simulink model "ThdRwRtStFwdBkwdIsPosChk"  (R2018b)
settings: Solver=FixedStepDiscrete  StartTime=0.0  StopTime=10.0  FixedStep=0.01  RelTol=1e-3
undefined symbols (not defined in the file or in its folder): KeSMSuThirdRwStFwdBkwdPosDelta_Val, KeSMSuThirdRwStFwdBkwdPosTolr_Val, KeSMSuVehicleModelConfig_Val
libraries: StIsPosChkLib x11, simulink x5
(part 1 of 2)
settings Model: Creator=sn2xws  LastModifiedBy=sn55gm
settings Model: ModifiedHistory=|
  | 2024.1.24
  | bug695362 7s 调用模式VIP R，3R无响应
  | 2024.3.14
  | V2.5.0
  | Bug 813950 童锁Lock，Mode1_Easy Entry Mode 不应调用失败
  | 2024.7.5 V3.0.0 557模式流程V1.9
  | 2024.8.28 V3.0.1 修改Lug干涉报成功逻辑
  | 2024.9.6 V3.0.2 新增Md56
  | 2024.10.14 V3.0.3新增Md57，Md58
  | 2024.11.11 V3.0.4 vip模式到位置不看三排
  | 2025.2.19 V3.8.0 Bug 991386 Md1 三排占座时未移动且报了成功
  | 25.7.1 V3.13.0 新增Md61 Md62
settings DataIOCC: SaveFormat=StructureWithTime
settings OptimizationCC: DefaultParameterBehavior=Inlined  EnhancedBackFolding=on  PassReuseOutputArgsAs=Individual arguments  ZeroExternalMemoryAtStartup=off  ZeroInternalMemoryAtStartup=off  OptimizeBlockOrder=speed  DifferentSizesBufferReuse=on  OptimizationCustomize=off
settings DebuggingCC: ParameterTunabilityLossMsg=error
settings ModelReferenceCC: ModelReferenceNumInstancesAllowed=Single
settings SFSimCC: MATLABDynamicMemAlloc=off
settings RTWCC: SystemTargetFile=autosar.tlc  GenCodeOnly=on  TemplateMakefile=ert_default_tmf  Description=AUTOSAR  GenerateReport=on  IncludeHyperlinkInReport=on  LaunchReport=on  GenerateTraceInfo=on  GenerateTraceReport=on  GenerateTraceReportSl=on  GenerateTraceReportSf=on  GenerateTraceReportEml=on
settings CodeAppCC: ForceParamTrailComments=on  IgnoreCustomStorageClasses=off  OperatorAnnotations=on  SimulinkDataObjDesc=on  SFDataObjDesc=on  InsertBlockDesc=on
settings STFCustomTargetCC: TargetLangStandard=C99 (ISO)  MultiwordLength=256  ParMdlRefBuildCompliant=on  CompOptLevelCompliant=on  IncludeMdlTerminateFcn=off  CombineOutputUpdateFcns=on  SuppressErrorStatus=on  ERTCustomFileBanners=on  SupportNonFinite=off  SupportComplex=off  SupportContinuousTime=off  SupportNonInlinedSFcns=off  RemoveResetFunc=on  MATLABClassNameForMDSCustomization=Simulink.SoftwareTarget.ERTCustomization  AutosarCompliant=on  UseToolchainInfoCompliant=on  LookupTableObjectStructAxisOrder=2,1,3,4,...  LUTObjectStructOrderEvenSpacing=Size,Table,Breakpoints  SystemTargetFile=autosar.tlc
settings ERTTargetCC: TargetLangStandard=C99 (ISO)  ConcurrentExecutionCompliant=off  IncludeMdlTerminateFcn=off  SuppressErrorStatus=on  SupportNonFinite=off  SupportComplex=off  ModelStepFunctionPrototypeControlCompliant=off  CPPClassGenCompliant=off  AutosarCompliant=on  LookupTableObjectStructAxisOrder=2,1,3,4,...  LUTObjectStructOrderEvenSpacing=Size,Table,Breakpoints  InlinedParameterPlacement=NonHierarchical  ERTCustomFileTemplate=example_file_process.tlc  ERTFilePackagingFormat=Compact

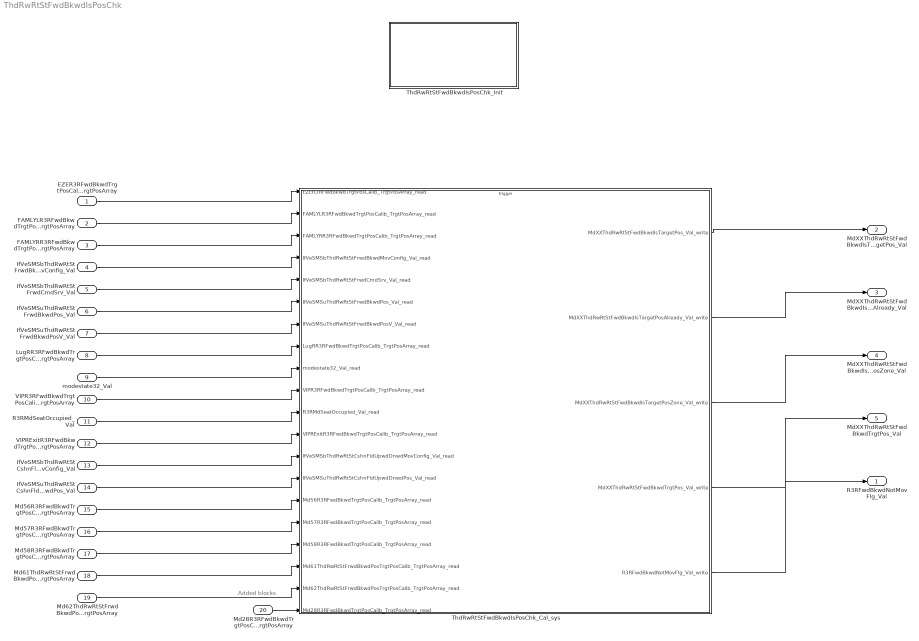
== system ThdRwRtStFwdBkwdIsPosChk ==
  note: Added blocks
  EZER3RFwdBkwdTrgtPosCalib_TrgtPosArray : Inport  Description=|  OutDataTypeStr=uint16  PortDimensions=3
      | 0:Pos
      | 1:Max
      | 2:Min
  FAMLYLR3RFwdBkwdTrgtPosCalib_TrgtPosArray : Inport  Description=|  Port=2  OutDataTypeStr=uint16  PortDimensions=3
      | 0:Pos
      | 1:Max
      | 2:Min
  FAMLYRR3RFwdBkwdTrgtPosCalib_TrgtPosArray : Inport  Description=|  Port=3  OutDataTypeStr=uint16  PortDimensions=3
      | 0:Pos
      | 1:Max
      | 2:Min
  IfVeSMSbThdRwRtStFrwdBkwdMovConfig_Val : Inport  Port=4  OutDataTypeStr=boolean  PortDimensions=1
  IfVeSMSbThdRwRtStFrwdCmdSrv_Val : Inport  Port=5  OutDataTypeStr=boolean  PortDimensions=1
  IfVeSMSuThdRwRtStFrwdBkwdPos_Val : Inport  Port=6  OutDataTypeStr=uint16  PortDimensions=1
  IfVeSMSuThdRwRtStFrwdBkwdPosV_Val : Inport  Port=7  OutDataTypeStr=boolean  PortDimensions=1
  LugRR3RFwdBkwdTrgtPosCalib_TrgtPosArray : Inport  Description=|  Port=8  OutDataTypeStr=uint16  PortDimensions=3
      | 0:Pos
      | 1:Max
      | 2:Min
  modestate32_Val : Inport  Port=9  OutDataTypeStr=uint32  PortDimensions=1
  VIPR3RFwdBkwdTrgtPosCalib_TrgtPosArray : Inport  Description=|  Port=10  OutDataTypeStr=uint16  PortDimensions=3
      | 0:Pos
      | 1:Max
      | 2:Min
  R3RMdSeatOccupied_Val : Inport  Port=11  OutDataTypeStr=boolean  PortDimensions=1
  VIPRExitR3RFwdBkwdTrgtPosCalib_TrgtPosArray : Inport  Description=|  Port=12  OutDataTypeStr=uint16  PortDimensions=3
      | 0:Pos
      | 1:Max
      | 2:Min
  IfVeSMSbThdRwRtStCshnFldUpwdDnwdMovConfig_Val : Inport  Port=13  OutDataTypeStr=boolean  PortDimensions=1
  IfVeSMSuThdRwRtStCshnFldUpwdDnwdPos_Val : Inport  Port=14  OutDataTypeStr=uint16  PortDimensions=1
  Md56R3RFwdBkwdTrgtPosCalib_TrgtPosArray : Inport  Description=|  Port=15  OutDataTypeStr=uint16  PortDimensions=3
      | 0:Pos
      | 1:Max
      | 2:Min
  Md57R3RFwdBkwdTrgtPosCalib_TrgtPosArray : Inport  Description=|  Port=16  OutDataTypeStr=uint16  PortDimensions=3
      | 0:Pos
      | 1:Max
      | 2:Min
  Md58R3RFwdBkwdTrgtPosCalib_TrgtPosArray : Inport  Description=|  Port=17  OutDataTypeStr=uint16  PortDimensions=3
      | 0:Pos
      | 1:Max
      | 2:Min
  Md61ThdRwRtStFrwdBkwdPosTrgtPosCalib_TrgtPosArray : Inport  Description=|  Port=18  OutDataTypeStr=uint16  PortDimensions=3
      | 0:Pos
      | 1:Max
      | 2:Min
  Md62ThdRwRtStFrwdBkwdPosTrgtPosCalib_TrgtPosArray : Inport  Description=|  Port=19  OutDataTypeStr=uint16  PortDimensions=3
      | 0:Pos
      | 1:Max
      | 2:Min
  Md28R3RFwdBkwdTrgtPosCalib_TrgtPosArray : Inport  Description=|  Port=20  OutDataTypeStr=uint16  PortDimensions=3
      | 0:Pos
      | 1:Max
      | 2:Min
  ThdRwRtStFwdBkwdIsPosChk_Cal_sys : Subsystem
  ThdRwRtStFwdBkwdIsPosChk_Init : Subsystem
  R3RFwdBkwdNotMovFlg_Val : Outport  OutDataTypeStr=boolean  PortDimensions=1
  MdXXThdRwRtStFwdBkwdIsTargetPos_Val : Outport  Port=2  OutDataTypeStr=uint32  PortDimensions=1
  MdXXThdRwRtStFwdBkwdIsTargetPosAlready_Val : Outport  Port=3  OutDataTypeStr=uint32  PortDimensions=1
  MdXXThdRwRtStFwdBkwdIsTargetPosZone_Val : Outport  Port=4  OutDataTypeStr=uint32  PortDimensions=1
  MdXXThdRwRtStFwdBkwdTrgtPos_Val : Outport  Port=5  OutDataTypeStr=uint16  PortDimensions=1
  wires:
  EZER3RFwdBkwdTrgtPosCalib_TrgtPosArray/1 -> ThdRwRtStFwdBkwdIsPosChk_Cal_sys/1(EZER3RFwdBkwdTrgtPosCalib_TrgtPosArray_read)
  FAMLYLR3RFwdBkwdTrgtPosCalib_TrgtPosArray/1 -> ThdRwRtStFwdBkwdIsPosChk_Cal_sys/2(FAMLYLR3RFwdBkwdTrgtPosCalib_TrgtPosArray_read)
  FAMLYRR3RFwdBkwdTrgtPosCalib_TrgtPosArray/1 -> ThdRwRtStFwdBkwdIsPosChk_Cal_sys/3(FAMLYRR3RFwdBkwdTrgtPosCalib_TrgtPosArray_read)
  IfVeSMSbThdRwRtStFrwdBkwdMovConfig_Val/1 -> ThdRwRtStFwdBkwdIsPosChk_Cal_sys/4(IfVeSMSbThdRwRtStFrwdBkwdMovConfig_Val_read)
  IfVeSMSbThdRwRtStFrwdCmdSrv_Val/1 -> ThdRwRtStFwdBkwdIsPosChk_Cal_sys/5(IfVeSMSbThdRwRtStFrwdCmdSrv_Val_read)
  IfVeSMSuThdRwRtStFrwdBkwdPos_Val/1 -> ThdRwRtStFwdBkwdIsPosChk_Cal_sys/6(IfVeSMSuThdRwRtStFrwdBkwdPos_Val_read)
  IfVeSMSuThdRwRtStFrwdBkwdPosV_Val/1 -> ThdRwRtStFwdBkwdIsPosChk_Cal_sys/7(IfVeSMSuThdRwRtStFrwdBkwdPosV_Val_read)
  LugRR3RFwdBkwdTrgtPosCalib_TrgtPosArray/1 -> ThdRwRtStFwdBkwdIsPosChk_Cal_sys/8(LugRR3RFwdBkwdTrgtPosCalib_TrgtPosArray_read)
  modestate32_Val/1 -> ThdRwRtStFwdBkwdIsPosChk_Cal_sys/9(modestate32_Val_read)
  VIPR3RFwdBkwdTrgtPosCalib_TrgtPosArray/1 -> ThdRwRtStFwdBkwdIsPosChk_Cal_sys/10(VIPR3RFwdBkwdTrgtPosCalib_TrgtPosArray_read)
  ThdRwRtStFwdBkwdIsPosChk_Cal_sys/1(MdXXThdRwRtStFwdBkwdIsTargetPos_Val_write) -> MdXXThdRwRtStFwdBkwdIsTargetPos_Val/1
  ThdRwRtStFwdBkwdIsPosChk_Cal_sys/2(MdXXThdRwRtStFwdBkwdIsTargetPosAlready_Val_write) -> MdXXThdRwRtStFwdBkwdIsTargetPosAlready_Val/1
  ThdRwRtStFwdBkwdIsPosChk_Cal_sys/3(MdXXThdRwRtStFwdBkwdIsTargetPosZone_Val_write) -> MdXXThdRwRtStFwdBkwdIsTargetPosZone_Val/1
  ThdRwRtStFwdBkwdIsPosChk_Cal_sys/4(MdXXThdRwRtStFwdBkwdTrgtPos_Val_write) -> MdXXThdRwRtStFwdBkwdTrgtPos_Val/1
  ThdRwRtStFwdBkwdIsPosChk_Cal_sys/5(R3RFwdBkwdNotMovFlg_Val_write) -> R3RFwdBkwdNotMovFlg_Val/1
  R3RMdSeatOccupied_Val/1 -> ThdRwRtStFwdBkwdIsPosChk_Cal_sys/11(R3RMdSeatOccupied_Val_read)
  VIPRExitR3RFwdBkwdTrgtPosCalib_TrgtPosArray/1 -> ThdRwRtStFwdBkwdIsPosChk_Cal_sys/12(VIPRExitR3RFwdBkwdTrgtPosCalib_TrgtPosArray_read)
  IfVeSMSbThdRwRtStCshnFldUpwdDnwdMovConfig_Val/1 -> ThdRwRtStFwdBkwdIsPosChk_Cal_sys/13(IfVeSMSbThdRwRtStCshnFldUpwdDnwdMovConfig_Val_read)
  IfVeSMSuThdRwRtStCshnFldUpwdDnwdPos_Val/1 -> ThdRwRtStFwdBkwdIsPosChk_Cal_sys/14(IfVeSMSuThdRwRtStCshnFldUpwdDnwdPos_Val_read)
  Md56R3RFwdBkwdTrgtPosCalib_TrgtPosArray/1 -> ThdRwRtStFwdBkwdIsPosChk_Cal_sys/15(Md56R3RFwdBkwdTrgtPosCalib_TrgtPosArray_read)
  Md57R3RFwdBkwdTrgtPosCalib_TrgtPosArray/1 -> ThdRwRtStFwdBkwdIsPosChk_Cal_sys/16(Md57R3RFwdBkwdTrgtPosCalib_TrgtPosArray_read)
  Md58R3RFwdBkwdTrgtPosCalib_TrgtPosArray/1 -> ThdRwRtStFwdBkwdIsPosChk_Cal_sys/17(Md58R3RFwdBkwdTrgtPosCalib_TrgtPosArray_read)
  Md61ThdRwRtStFrwdBkwdPosTrgtPosCalib_TrgtPosArray/1 -> ThdRwRtStFwdBkwdIsPosChk_Cal_sys/18(Md61ThdRwRtStFrwdBkwdPosTrgtPosCalib_TrgtPosArray_read)
  Md62ThdRwRtStFrwdBkwdPosTrgtPosCalib_TrgtPosArray/1 -> ThdRwRtStFwdBkwdIsPosChk_Cal_sys/19(Md62ThdRwRtStFrwdBkwdPosTrgtPosCalib_TrgtPosArray_read)
  Md28R3RFwdBkwdTrgtPosCalib_TrgtPosArray/1 -> ThdRwRtStFwdBkwdIsPosChk_Cal_sys/20(Md28R3RFwdBkwdTrgtPosCalib_TrgtPosArray_read)

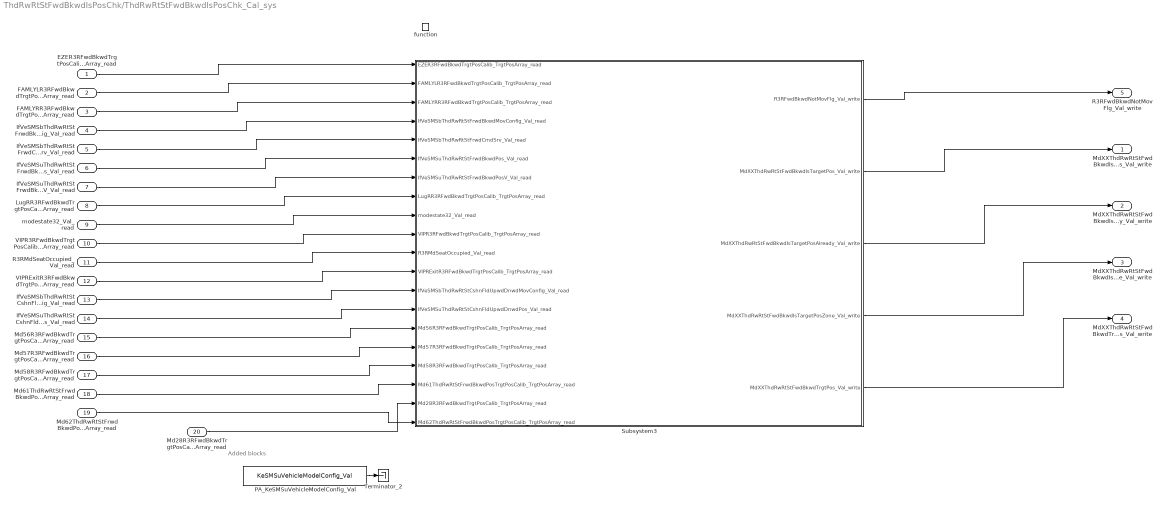
== system ThdRwRtStFwdBkwdIsPosChk/ThdRwRtStFwdBkwdIsPosChk_Cal_sys ==
  note: Added blocks
  EZER3RFwdBkwdTrgtPosCalib_TrgtPosArray_read : Inport
  FAMLYLR3RFwdBkwdTrgtPosCalib_TrgtPosArray_read : Inport  Port=2
  FAMLYRR3RFwdBkwdTrgtPosCalib_TrgtPosArray_read : Inport  Port=3
  IfVeSMSbThdRwRtStFrwdBkwdMovConfig_Val_read : Inport  Port=4
  IfVeSMSbThdRwRtStFrwdCmdSrv_Val_read : Inport  Port=5
  IfVeSMSuThdRwRtStFrwdBkwdPos_Val_read : Inport  Port=6
  IfVeSMSuThdRwRtStFrwdBkwdPosV_Val_read : Inport  Port=7
  LugRR3RFwdBkwdTrgtPosCalib_TrgtPosArray_read : Inport  Port=8
  modestate32_Val_read : Inport  Port=9
  VIPR3RFwdBkwdTrgtPosCalib_TrgtPosArray_read : Inport  Port=10
  R3RMdSeatOccupied_Val_read : Inport  Port=11
  VIPRExitR3RFwdBkwdTrgtPosCalib_TrgtPosArray_read : Inport  Port=12
  IfVeSMSbThdRwRtStCshnFldUpwdDnwdMovConfig_Val_read : Inport  Port=13
  IfVeSMSuThdRwRtStCshnFldUpwdDnwdPos_Val_read : Inport  Port=14
  Md56R3RFwdBkwdTrgtPosCalib_TrgtPosArray_read : Inport  Port=15
  Md57R3RFwdBkwdTrgtPosCalib_TrgtPosArray_read : Inport  Port=16
  Md58R3RFwdBkwdTrgtPosCalib_TrgtPosArray_read : Inport  Port=17
  Md61ThdRwRtStFrwdBkwdPosTrgtPosCalib_TrgtPosArray_read : Inport  Port=18
  Md62ThdRwRtStFrwdBkwdPosTrgtPosCalib_TrgtPosArray_read : Inport  Port=19
  Md28R3RFwdBkwdTrgtPosCalib_TrgtPosArray_read : Inport  Port=20
  function : TriggerPort  TriggerType=function-call  IsSimulinkFunction=on  FunctionName=ThdRwRtStFwdBkwdIsPosChk_Cal  VariantControl=(inherit)
  PA_KeSMSuVehicleModelConfig_Val : Constant  Value=KeSMSuVehicleModelConfig_Val
  Subsystem3 : Subsystem
  Terminator_2 : Terminator
  MdXXThdRwRtStFwdBkwdIsTargetPos_Val_write : Outport
      settings: EnsureOutportIsVirtual=on
  MdXXThdRwRtStFwdBkwdIsTargetPosAlready_Val_write : Outport  Port=2
      settings: EnsureOutportIsVirtual=on
  MdXXThdRwRtStFwdBkwdIsTargetPosZone_Val_write : Outport  Port=3
      settings: EnsureOutportIsVirtual=on
  MdXXThdRwRtStFwdBkwdTrgtPos_Val_write : Outport  Port=4
      settings: EnsureOutportIsVirtual=on
  R3RFwdBkwdNotMovFlg_Val_write : Outport  Port=5
      settings: EnsureOutportIsVirtual=on
  wires:
  Subsystem3/2(MdXXThdRwRtStFwdBkwdIsTargetPos_Val_write) -> MdXXThdRwRtStFwdBkwdIsTargetPos_Val_write/1
  Subsystem3/3(MdXXThdRwRtStFwdBkwdIsTargetPosAlready_Val_write) -> MdXXThdRwRtStFwdBkwdIsTargetPosAlready_Val_write/1
  Subsystem3/1(R3RFwdBkwdNotMovFlg_Val_write) -> R3RFwdBkwdNotMovFlg_Val_write/1
  Subsystem3/4(MdXXThdRwRtStFwdBkwdIsTargetPosZone_Val_write) -> MdXXThdRwRtStFwdBkwdIsTargetPosZone_Val_write/1
  Subsystem3/5(MdXXThdRwRtStFwdBkwdTrgtPos_Val_write) -> MdXXThdRwRtStFwdBkwdTrgtPos_Val_write/1
  EZER3RFwdBkwdTrgtPosCalib_TrgtPosArray_read/1 -> Subsystem3/1(EZER3RFwdBkwdTrgtPosCalib_TrgtPosArray_read)
  FAMLYLR3RFwdBkwdTrgtPosCalib_TrgtPosArray_read/1 -> Subsystem3/2(FAMLYLR3RFwdBkwdTrgtPosCalib_TrgtPosArray_read)
  FAMLYRR3RFwdBkwdTrgtPosCalib_TrgtPosArray_read/1 -> Subsystem3/3(FAMLYRR3RFwdBkwdTrgtPosCalib_TrgtPosArray_read)
  IfVeSMSbThdRwRtStFrwdBkwdMovConfig_Val_read/1 -> Subsystem3/4(IfVeSMSbThdRwRtStFrwdBkwdMovConfig_Val_read)
  IfVeSMSbThdRwRtStFrwdCmdSrv_Val_read/1 -> Subsystem3/5(IfVeSMSbThdRwRtStFrwdCmdSrv_Val_read)
  IfVeSMSuThdRwRtStFrwdBkwdPos_Val_read/1 -> Subsystem3/6(IfVeSMSuThdRwRtStFrwdBkwdPos_Val_read)
  IfVeSMSuThdRwRtStFrwdBkwdPosV_Val_read/1 -> Subsystem3/7(IfVeSMSuThdRwRtStFrwdBkwdPosV_Val_read)
  LugRR3RFwdBkwdTrgtPosCalib_TrgtPosArray_read/1 -> Subsystem3/8(LugRR3RFwdBkwdTrgtPosCalib_TrgtPosArray_read)
  modestate32_Val_read/1 -> Subsystem3/9(modestate32_Val_read)
  VIPR3RFwdBkwdTrgtPosCalib_TrgtPosArray_read/1 -> Subsystem3/10(VIPR3RFwdBkwdTrgtPosCalib_TrgtPosArray_read)
  R3RMdSeatOccupied_Val_read/1 -> Subsystem3/11(R3RMdSeatOccupied_Val_read)
  VIPRExitR3RFwdBkwdTrgtPosCalib_TrgtPosArray_read/1 -> Subsystem3/12(VIPRExitR3RFwdBkwdTrgtPosCalib_TrgtPosArray_read)
  IfVeSMSbThdRwRtStCshnFldUpwdDnwdMovConfig_Val_read/1 -> Subsystem3/13(IfVeSMSbThdRwRtStCshnFldUpwdDnwdMovConfig_Val_read)
  IfVeSMSuThdRwRtStCshnFldUpwdDnwdPos_Val_read/1 -> Subsystem3/14(IfVeSMSuThdRwRtStCshnFldUpwdDnwdPos_Val_read)
  Md56R3RFwdBkwdTrgtPosCalib_TrgtPosArray_read/1 -> Subsystem3/15(Md56R3RFwdBkwdTrgtPosCalib_TrgtPosArray_read)
  Md57R3RFwdBkwdTrgtPosCalib_TrgtPosArray_read/1 -> Subsystem3/16(Md57R3RFwdBkwdTrgtPosCalib_TrgtPosArray_read)
  Md58R3RFwdBkwdTrgtPosCalib_TrgtPosArray_read/1 -> Subsystem3/17(Md58R3RFwdBkwdTrgtPosCalib_TrgtPosArray_read)
  Md61ThdRwRtStFrwdBkwdPosTrgtPosCalib_TrgtPosArray_read/1 -> Subsystem3/18(Md61ThdRwRtStFrwdBkwdPosTrgtPosCalib_TrgtPosArray_read)
  Md62ThdRwRtStFrwdBkwdPosTrgtPosCalib_TrgtPosArray_read/1 -> Subsystem3/20(Md62ThdRwRtStFrwdBkwdPosTrgtPosCalib_TrgtPosArray_read)
  Md28R3RFwdBkwdTrgtPosCalib_TrgtPosArray_read/1 -> Subsystem3/19(Md28R3RFwdBkwdTrgtPosCalib_TrgtPosArray_read)
  PA_KeSMSuVehicleModelConfig_Val/1 -> Terminator_2/1

== system ThdRwRtStFwdBkwdIsPosChk/ThdRwRtStFwdBkwdIsPosChk_Init ==
  note: Added blocks
  note: Added blocks
  note: Added blocks
  Event Listener : EventListener  EventName=reset
  PA_KeSMSuThirdRwStFwdBkwdPosDelta_Val : Constant  Value=KeSMSuThirdRwStFwdBkwdPosDelta_Val
  PA_KeSMSuThirdRwStFwdBkwdPosTolr_Val : Constant  Value=KeSMSuThirdRwStFwdBkwdPosTolr_Val
  PA_KeSMSuVehicleModelConfig_Val : Constant  Value=KeSMSuVehicleModelConfig_Val
  Terminator_1 : Terminator
  Terminator_2 : Terminator
  Terminator_3 : Terminator
  wires:
  PA_KeSMSuThirdRwStFwdBkwdPosDelta_Val/1 -> Terminator_1/1
  PA_KeSMSuThirdRwStFwdBkwdPosTolr_Val/1 -> Terminator_2/1
  PA_KeSMSuVehicleModelConfig_Val/1 -> Terminator_3/1

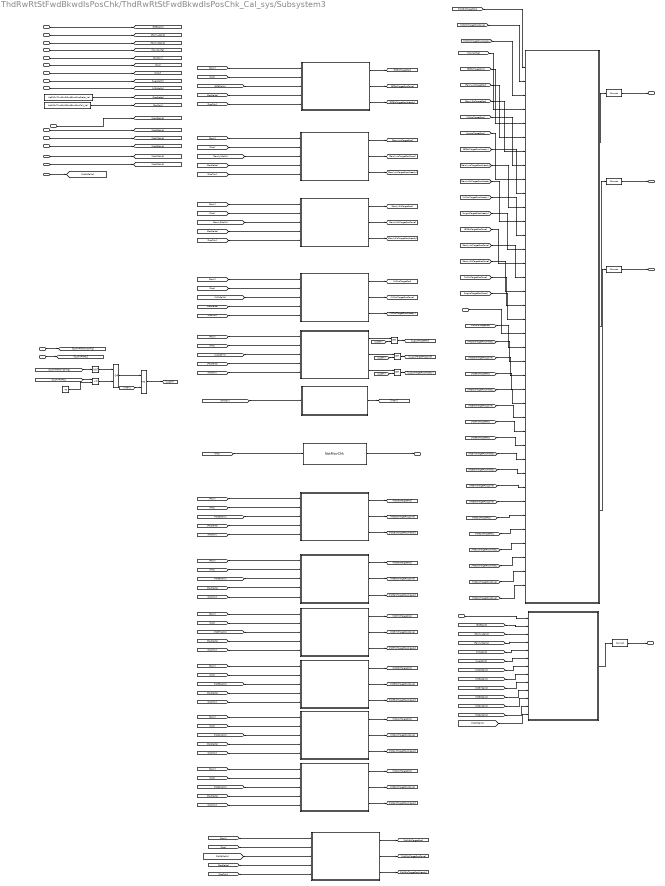
== system ThdRwRtStFwdBkwdIsPosChk/ThdRwRtStFwdBkwdIsPosChk_Cal_sys/Subsystem3 ==
  note: 增加Lug模式如果没有发生干涉但是到了最前面也算成功
  EZER3RFwdBkwdTrgtPosCalib_TrgtPosArray_read : Inport
  FAMLYLR3RFwdBkwdTrgtPosCalib_TrgtPosArray_read : Inport  Port=2
  FAMLYRR3RFwdBkwdTrgtPosCalib_TrgtPosArray_read : Inport  Port=3
  IfVeSMSbThdRwRtStFrwdBkwdMovConfig_Val_read : Inport  Port=4
  IfVeSMSbThdRwRtStFrwdCmdSrv_Val_read : Inport  Port=5
  IfVeSMSuThdRwRtStFrwdBkwdPos_Val_read : Inport  Port=6
  IfVeSMSuThdRwRtStFrwdBkwdPosV_Val_read : Inport  Port=7
  LugRR3RFwdBkwdTrgtPosCalib_TrgtPosArray_read : Inport  Port=8
  modestate32_Val_read : Inport  Port=9
  VIPR3RFwdBkwdTrgtPosCalib_TrgtPosArray_read : Inport  Port=10
  R3RMdSeatOccupied_Val_read : Inport  Port=11
  VIPRExitR3RFwdBkwdTrgtPosCalib_TrgtPosArray_read : Inport  Port=12
  IfVeSMSbThdRwRtStCshnFldUpwdDnwdMovConfig_Val_read : Inport  Port=13
  IfVeSMSuThdRwRtStCshnFldUpwdDnwdPos_Val_read : Inport  Port=14
  Md56R3RFwdBkwdTrgtPosCalib_TrgtPosArray_read : Inport  Port=15
  Md57R3RFwdBkwdTrgtPosCalib_TrgtPosArray_read : Inport  Port=16
  Md58R3RFwdBkwdTrgtPosCalib_TrgtPosArray_read : Inport  Port=17
  Md61ThdRwRtStFrwdBkwdPosTrgtPosCalib_TrgtPosArray_read : Inport  Port=18
  Md28R3RFwdBkwdTrgtPosCalib_TrgtPosArray_read : Inport  Port=19
  Md62ThdRwRtStFrwdBkwdPosTrgtPosCalib_TrgtPosArray_read : Inport  Port=20
  Constant : Constant  Value=40  OutDataTypeStr=uint16
  Data Type Conversion{,1..3} (4 alike) : DataTypeConversion
  Logical Operator{,1,4..5} (4 alike) : Logic  Operator=OR  AllPortsSameDT=off  OutDataTypeStr=boolean
  Logical Operator2 : Logic  Operator=NOT  AllPortsSameDT=off  OutDataTypeStr=boolean
  Logical Operator3 : Logic  AllPortsSameDT=off  OutDataTypeStr=boolean
  NotMovChk : StIsPosChkLib/NotMovChk  SystemSampleTime=-1
  PA_KeSMSuThirdRwStFwdBkwdPosDelta_Val : Constant  Value=KeSMSuThirdRwStFwdBkwdPosDelta_Val
  PA_KeSMSuThirdRwStFwdBkwdPosTolr_Val : Constant  Value=KeSMSuThirdRwStFwdBkwdPosTolr_Val
  Relational Operator : RelationalOperator  Operator=<=  OutDataTypeStr=boolean  RndMeth=Simplest
  Subsystem : Subsystem
  Subsystem1 : Subsystem
  Subsystem10 : Subsystem
  Subsystem11 : Subsystem
  Subsystem12 : Subsystem
  Subsystem13 : Subsystem
  Subsystem14 : Subsystem
  Subsystem2 : Subsystem
  Subsystem3 : Subsystem
  Subsystem4 : Subsystem
  Subsystem5 : Subsystem
  Subsystem6 : Subsystem
  Subsystem7 : Subsystem
  Subsystem8 : Subsystem
  Subsystem9 : Subsystem
  R3RFwdBkwdNotMovFlg_Val_write : Outport
      settings: EnsureOutportIsVirtual=on
  MdXXThdRwRtStFwdBkwdIsTargetPos_Val_write : Outport  Port=2
      settings: EnsureOutportIsVirtual=on
  MdXXThdRwRtStFwdBkwdIsTargetPosAlready_Val_write : Outport  Port=3
      settings: EnsureOutportIsVirtual=on
  MdXXThdRwRtStFwdBkwdIsTargetPosZone_Val_write : Outport  Port=4
      settings: EnsureOutportIsVirtual=on
  MdXXThdRwRtStFwdBkwdTrgtPos_Val_write : Outport  Port=5
      settings: EnsureOutportIsVirtual=on
  wires:
  [PosV] -> Subsystem5/1(PosV)
  Subsystem3/3(IsPosAlready) -> [FamlyLIsTargetPosAlready]
  Subsystem1/1(IsTargetPos) -> Data Type Conversion1/1
  [Pos] -> Subsystem5/2(Pos)
  Subsystem/1(TrgtPos) -> Data Type Conversion/1
  [VIPLIsTargetPosAlready] -> Subsystem1/13(VIPLIsTargetPosAlready)
  [PosV] -> Subsystem4/1(PosV)
  IfVeSMSuThdRwRtStFrwdBkwdPosV_Val_read/1 -> [PosV]
  [LugLCalib] -> Subsystem/6(LugLCalib)
  Subsystem3/1(IsPos) -> [FamlyLIsTargetPos]
  FAMLYLR3RFwdBkwdTrgtPosCalib_TrgtPosArray_read/1 -> [FamlyLCalib]
  EZER3RFwdBkwdTrgtPosCalib_TrgtPosArray_read/1 -> [EZECalib]
  [EZEIsTargetPosZone] -> Subsystem1/15(EZEIsTargetPosZone)
  [PosDelta] -> Subsystem5/4(Delta)
  [Pos] -> Subsystem6/2(Pos)
  VIPR3RFwdBkwdTrgtPosCalib_TrgtPosArray_read/1 -> [VIPLCalib]
  [FamlyRIsTargetPosAlready] -> Subsystem1/12(FamlyRIsTargetPosAlready)
  [PosV] -> Subsystem6/1(PosV)
  [PosDelta] -> Subsystem4/4(Delta)
  [MovConfig] -> Subsystem1/4(MovConfig)
  [EZEIsTargetPosAlready] -> Subsystem1/10(EZEIsTargetPosAlready)
  Subsystem5/2(IsPosZone) -> [FamlyRIsTargetPosZone]
  IfVeSMSbThdRwRtStFrwdCmdSrv_Val_read/1 -> [CmdSrv]
  [PosV] -> Subsystem3/1(PosV)
  [FamlyLIsTargetPosZone] -> Subsystem1/16(FamlyLIsTargetPosZone)
  [PosTolr] -> Subsystem6/5(Tolr)
  Subsystem1/3(IsTargetPosZone) -> Data Type Conversion3/1
  [FamlyLIsTargetPos] -> Subsystem1/6(FamlyLIsTargetPos)
  [EZEIsTargetPos] -> Subsystem1/5(EZEIsTargetPos)
  [Pos] -> Subsystem3/2(Pos)
  [VIPLIsTargetPosZone] -> Subsystem1/18(VIPLIsTargetPosZone)
  [LugLIsTargetPos] -> Subsystem1/9(INTMLIsTargetPos)
  [VIPLCalib] -> Subsystem6/3(CalibArray)
  PA_KeSMSuThirdRwStFwdBkwdPosTolr_Val/1 -> [PosTolr]
  Subsystem6/3(IsPosAlready) -> [VIPLIsTargetPosAlready]
  [EZECalib] -> Subsystem4/3(CalibArray)
  IfVeSMSbThdRwRtStFrwdBkwdMovConfig_Val_read/1 -> [MovConfig]
  FAMLYRR3RFwdBkwdTrgtPosCalib_TrgtPosArray_read/1 -> [FamlyRCalib]
  [VIPLCalib] -> Subsystem/5(VIPLCalib)
  Subsystem6/2(IsPosZone) -> [VIPLIsTargetPosZone]
  [CmdSrv] -> Subsystem2/1(CmdSrv)
  Subsystem5/3(IsPosAlready) -> [FamlyRIsTargetPosAlready]
  LugRR3RFwdBkwdTrgtPosCalib_TrgtPosArray_read/1 -> [LugLCalib]
  Subsystem5/1(IsPos) -> [FamlyRIsTargetPos]
  [PosDelta] -> Subsystem3/4(Delta)
  PA_KeSMSuThirdRwStFwdBkwdPosDelta_Val/1 -> [PosDelta]
  Subsystem6/1(IsPos) -> [VIPLIsTargetPos]
  Data Type Conversion2/1 -> MdXXThdRwRtStFwdBkwdIsTargetPosAlready_Val_write/1
  Subsystem1/2(IsTargetPosAlready) -> Data Type Conversion2/1
  [PosTolr] -> Subsystem4/5(Tolr)
  [VIPLIsTargetPos] -> Subsystem1/8(VIPLIsTargetPos)
  [FamlyLCalib] -> Subsystem3/3(CalibArray)
  [FamlyLCalib] -> Subsystem/3(FamlyLCalib)
  [EZECalib] -> Subsystem/2(EZECalib)
  Subsystem4/3(IsPosAlready) -> [EZEIsTargetPosAlready]
  NotMovChk/1 -> R3RFwdBkwdNotMovFlg_Val_write/1
  [Pos] -> NotMovChk/1
  [FamlyRIsTargetPos] -> Subsystem1/7(FamlyRIsTargetPos)
  Subsystem4/1(IsPos) -> [EZEIsTargetPos]
  [PosDelta] -> Subsystem6/4(Delta)
  [LugLIsTargetPosAlready] -> Subsystem1/14(INTMLIsTargetPosAlready)
  [FamlyRCalib] -> Subsystem/4(FamlyRCalib)
  Subsystem3/2(IsPosZone) -> [FamlyLIsTargetPosZone]
  [Pos] -> Subsystem4/2(Pos)
  [LugLIsTargetPosZone] -> Subsystem1/19(INTMLIsTargetPosZone)
  IfVeSMSuThdRwRtStFrwdBkwdPos_Val_read/1 -> [Pos]
  Data Type Conversion3/1 -> MdXXThdRwRtStFwdBkwdIsTargetPosZone_Val_write/1
  [FamlyRCalib] -> Subsystem5/3(CalibArray)
  modestate32_Val_read/1 -> Subsystem/1(modestate32_Val_read)
  [FamlyRIsTargetPosZone] -> Subsystem1/17(FamlyRIsTargetPosZone)
  Subsystem4/2(IsPosZone) -> [EZEIsTargetPosZone]
  [FamlyLIsTargetPosAlready] -> Subsystem1/11(FamlyLIsTargetPosAlready)
  Data Type Conversion1/1 -> MdXXThdRwRtStFwdBkwdIsTargetPos_Val_write/1
  [PosTolr] -> Subsystem5/5(Tolr)
  [PosTolr] -> Subsystem3/5(Tolr)
  Data Type Conversion/1 -> MdXXThdRwRtStFwdBkwdTrgtPos_Val_write/1
  [PosDelta] -> Subsystem7/4(Delta)
  [LugLCalib] -> Subsystem7/3(CalibArray)
  [PosTolr] -> Subsystem7/5(Tolr)
  [PosV] -> Subsystem7/1(PosV)
  [Pos] -> Subsystem7/2(Pos)
  Subsystem2/1(IsTargetPos) -> [interv]
  Logical Operator1/1 -> [LugLIsTargetPosZone]
  Subsystem7/2(IsPosZone) -> Logical Operator1/1
  [LugOK] -> Logical Operator1/2
  R3RMdSeatOccupied_Val_read/1 -> Subsystem1/20(R3RMdSeatOccupied_Val_read)
  [PosDelta] -> Subsystem8/4(Delta)
  Subsystem8/1(IsPos) -> [Md28IsTargetPos]
  Subsystem8/2(IsPosZone) -> [Md28IsTargetPosZone]
  Subsystem8/3(IsPosAlready) -> [Md28IsTargetPosAlready]
  [Md28Calib] -> Subsystem8/3(CalibArray)
  [PosTolr] -> Subsystem8/5(Tolr)
  [PosV] -> Subsystem8/1(PosV)
  [Pos] -> Subsystem8/2(Pos)
  [Md28Calib] -> Subsystem/7(Md28Calib)
  [Md28IsTargetPosZone] -> Subsystem1/23(Md28IsTargetPosZone)
  [Md28IsTargetPosAlready] -> Subsystem1/22(Md28IsTargetPosAlready)
  [Md28IsTargetPos] -> Subsystem1/21(Md28IsTargetPos)
  Constant/1 -> Relational Operator/2
  Logical Operator2/1 -> Logical Operator/1
  [CushnFldPos] -> Relational Operator/1
  [CushnFldMovConfig] -> Logical Operator2/1
  [interv] -> Logical Operator3/2
  Relational Operator/1 -> Logical Operator/2
  Logical Operator/1 -> Logical Operator3/1
  Logical Operator3/1 -> [LugOK]
  IfVeSMSbThdRwRtStCshnFldUpwdDnwdMovConfig_Val_read/1 -> [CushnFldMovConfig]
  IfVeSMSuThdRwRtStCshnFldUpwdDnwdPos_Val_read/1 -> [CushnFldPos]
  Logical Operator4/1 -> [LugLIsTargetPos]
  Subsystem7/1(IsPos) -> Logical Operator4/1
  [LugOK] -> Logical Operator4/2
  Logical Operator5/1 -> [LugLIsTargetPosAlready]
  Subsystem7/3(IsPosAlready) -> Logical Operator5/1
  [LugOK] -> Logical Operator5/2
  Md56R3RFwdBkwdTrgtPosCalib_TrgtPosArray_read/1 -> [Md56Calib]
  [Md56Calib] -> Subsystem/8(Md56Calib)
  [Pos] -> Subsystem9/2(Pos)
  [PosV] -> Subsystem9/1(PosV)
  [PosTolr] -> Subsystem9/5(Tolr)
  [Md56Calib] -> Subsystem9/3(CalibArray)
  Subsystem9/3(IsPosAlready) -> [Md56IsTargetPosAlready]
  Subsystem9/2(IsPosZone) -> [Md56IsTargetPosZone]
  Subsystem9/1(IsPos) -> [Md56IsTargetPos]
  [PosDelta] -> Subsystem9/4(Delta)
  [Md56IsTargetPos] -> Subsystem1/24(Md56IsTargetPos)
  [Md56IsTargetPosAlready] -> Subsystem1/25(Md56IsTargetPosAlready)
  [Md56IsTargetPosZone] -> Subsystem1/26(Md56IsTargetPosZone)
  Md58R3RFwdBkwdTrgtPosCalib_TrgtPosArray_read/1 -> [Md58Calib]
  Md57R3RFwdBkwdTrgtPosCalib_TrgtPosArray_read/1 -> [Md57Calib]
  [PosDelta] -> Subsystem10/4(Delta)
  Subsystem10/1(IsPos) -> [Md57IsTargetPos]
  Subsystem10/2(IsPosZone) -> [Md57IsTargetPosZone]
  Subsystem10/3(IsPosAlready) -> [Md57IsTargetPosAlready]
  [Md57Calib] -> Subsystem10/3(CalibArray)
  [PosTolr] -> Subsystem10/5(Tolr)
  [PosV] -> Subsystem10/1(PosV)
  [Pos] -> Subsystem10/2(Pos)
  [Pos] -> Subsystem11/2(Pos)
  [PosV] -> Subsystem11/1(PosV)
  [PosTolr] -> Subsystem11/5(Tolr)
  [Md58Calib] -> Subsystem11/3(CalibArray)
  Subsystem11/3(IsPosAlready) -> [Md58IsTargetPosAlready]
  Subsystem11/2(IsPosZone) -> [Md58IsTargetPosZone]
  Subsystem11/1(IsPos) -> [Md58IsTargetPos]
  [PosDelta] -> Subsystem11/4(Delta)
  [Md58Calib] -> Subsystem/10(Md58Calib)
  [Md57Calib] -> Subsystem/9(Md57Calib)
  [Md58IsTargetPos] -> Subsystem1/28(Md58IsTargetPos)
  [Md57IsTargetPos] -> Subsystem1/27(Md57IsTargetPos)
  [Md57IsTargetPosAlready] -> Subsystem1/29(Md57IsTargetPosAlready)
  [Md58IsTargetPosAlready] -> Subsystem1/30(Md58IsTargetPosAlready)
  [Md57IsTargetPosZone] -> Subsystem1/31(Md57IsTargetPosZone)
  [Md58IsTargetPosZone] -> Subsystem1/32(Md58IsTargetPosZone)
  Md62ThdRwRtStFrwdBkwdPosTrgtPosCalib_TrgtPosArray_read/1 -> [Md62Calib]
  Md61ThdRwRtStFrwdBkwdPosTrgtPosCalib_TrgtPosArray_read/1 -> [Md61Calib]
  [PosDelta] -> Subsystem12/4(Delta)
  Subsystem12/1(IsPos) -> [Md61IsTargetPos]
  Subsystem12/2(IsPosZone) -> [Md61IsTargetPosZone]
  Subsystem12/3(IsPosAlready) -> [Md61IsTargetPosAlready]
  [Md61Calib] -> Subsystem12/3(CalibArray)
  [PosTolr] -> Subsystem12/5(Tolr)
  [PosV] -> Subsystem12/1(PosV)
  [Pos] -> Subsystem12/2(Pos)
  [Pos] -> Subsystem13/2(Pos)
  [PosV] -> Subsystem13/1(PosV)
  [PosTolr] -> Subsystem13/5(Tolr)
  [Md62Calib] -> Subsystem13/3(CalibArray)
  Subsystem13/3(IsPosAlready) -> [Md62IsTargetPosAlready]
  Subsystem13/2(IsPosZone) -> [Md62IsTargetPosZone]
  Subsystem13/1(IsPos) -> [Md62IsTargetPos]
  [PosDelta] -> Subsystem13/4(Delta)
  [Md61Calib] -> Subsystem/11(Md61Calib)
  [Md62Calib] -> Subsystem/12(Md62Calib)
  [Md61IsTargetPos] -> Subsystem1/33(Md61IsTargetPos)
  [Md62IsTargetPos] -> Subsystem1/34(Md62IsTargetPos)
  [Md62IsTargetPosZone] -> Subsystem1/38(Md62IsTargetPosZone)
  [Md61IsTargetPosZone] -> Subsystem1/37(Md61IsTargetPosZone)
  [Md62IsTargetPosAlready] -> Subsystem1/36(Md62IsTargetPosAlready)
  [Md61IsTargetPosAlready] -> Subsystem1/35(Md61IsTargetPosAlready)
  VIPRExitR3RFwdBkwdTrgtPosCalib_TrgtPosArray_read/1 -> [Md28Calib]
  Md28R3RFwdBkwdTrgtPosCalib_TrgtPosArray_read/1 -> [Md15Calib]
  Subsystem14/2(IsPosZone) -> [Md15IsTargetPosZone]
  Subsystem14/3(IsPosAlready) -> [Md15IsTargetPosAlready]
  Subsystem14/1(IsPos) -> [Md15IsTargetPos]
  [PosV] -> Subsystem14/1(PosV)
  [Md15Calib] -> Subsystem14/3(CalibArray)
  [PosTolr] -> Subsystem14/5(Tolr)
  [PosDelta] -> Subsystem14/4(Delta)
  [Pos] -> Subsystem14/2(Pos)
  [Md15IsTargetPosAlready] -> Subsystem1/3(Md15IsTargetPosAlready)
  [Md15IsTargetPosZone] -> Subsystem1/2(Md15IsTargetPosZone)
  [Md15IsTargetPos] -> Subsystem1/1(Md15IsTargetPos)
  [Md15Calib] -> Subsystem/13(Md15Calib)

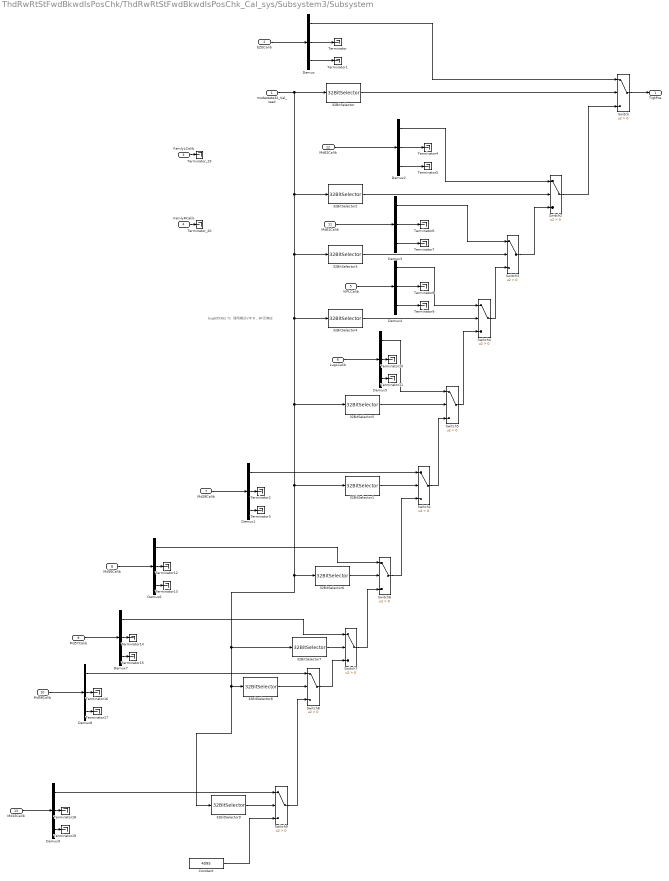
== system ThdRwRtStFwdBkwdIsPosChk/ThdRwRtStFwdBkwdIsPosChk_Cal_sys/Subsystem3/Subsystem ==
  note: bug695362 7s 调用模式VIP R，3R无响应
  modestate32_Val_read : Inport
  EZECalib : Inport  Port=2
  FamlyLCalib : Inport  Port=3
  FamlyRCalib : Inport  Port=4
  VIPLCalib : Inport  Port=5
  LugLCalib : Inport  Port=6
  Md28Calib : Inport  Port=7
  Md56Calib : Inport  Port=8
  Md57Calib : Inport  Port=9
  Md58Calib : Inport  Port=10
  Md61Calib : Inport  Port=11
  Md62Calib : Inport  Port=12
  Md15Calib : Inport  Port=13
  32BitSelector : StIsPosChkLib/32BitSelector  BitNum=0
  32BitSelector1 : StIsPosChkLib/32BitSelector  BitNum=27
  32BitSelector2 : StIsPosChkLib/32BitSelector  BitNum=6
  32BitSelector3 : StIsPosChkLib/32BitSelector  BitNum=5
  32BitSelector4 : StIsPosChkLib/32BitSelector  BitNum=11
  32BitSelector5 : StIsPosChkLib/32BitSelector  BitNum=8
  32BitSelector6 : StIsPosChkLib/32BitSelector  BitNum=24
  32BitSelector7 : StIsPosChkLib/32BitSelector  BitNum=20
  32BitSelector8 : StIsPosChkLib/32BitSelector  BitNum=21
  32BitSelector9 : StIsPosChkLib/32BitSelector  BitNum=14
  Constant : Constant  Value=4095  OutDataTypeStr=uint16
  Demux{,1..9} (10 alike) : Demux  Outputs=3
  Switch{,1..9} (10 alike) : Switch  Criteria=u2 > Threshold
  Terminator{,1..19} (20 alike) : Terminator
  Terminator_19 : Terminator
  Terminator_20 : Terminator
  TrgtPos : Outport
      settings: EnsureOutportIsVirtual=on
  wires:
  32BitSelector/1 -> Switch/2
  Demux/1 -> Switch/1
  Demux/3 -> Terminator1/1
  Demux/2 -> Terminator/1
  EZECalib/1 -> Demux/1
  Switch/1 -> TrgtPos/1
  Switch2/1 -> Switch/3
  Switch3/1 -> Switch2/3
  Switch4/1 -> Switch3/3
  32BitSelector2/1 -> Switch2/2
  32BitSelector3/1 -> Switch3/2
  32BitSelector4/1 -> Switch4/2
  Demux2/1 -> Switch2/1
  Demux2/3 -> Terminator5/1
  Demux2/2 -> Terminator4/1
  Demux3/2 -> Terminator6/1
  Demux3/3 -> Terminator7/1
  Demux3/1 -> Switch3/1
  Demux4/1 -> Switch4/1
  Demux4/3 -> Terminator9/1
  Demux4/2 -> Terminator8/1
  VIPLCalib/1 -> Demux4/1
  LugLCalib/1 -> Demux5/1
  Demux5/2 -> Terminator10/1
  Demux5/3 -> Terminator11/1
  Demux5/1 -> Switch5/1
  32BitSelector5/1 -> Switch5/2
  Switch5/1 -> Switch4/3
  Demux1/1 -> Switch1/1
  Demux1/3 -> Terminator3/1
  Demux1/2 -> Terminator2/1
  Md28Calib/1 -> Demux1/1
  Switch1/1 -> Switch5/3
  32BitSelector1/1 -> Switch1/2
  Switch6/1 -> Switch1/3
  32BitSelector6/1 -> Switch6/2
  Md56Calib/1 -> Demux6/1
  Demux6/2 -> Terminator12/1
  Demux6/3 -> Terminator13/1
  Demux6/1 -> Switch6/1
  Switch7/1 -> Switch6/3
  Switch8/1 -> Switch7/3
  32BitSelector7/1 -> Switch7/2
  32BitSelector8/1 -> Switch8/2
  modestate32_Val_read/1 -> 32BitSelector2/1, 32BitSelector5/1, 32BitSelector7/1, 32BitSelector9/1, 32BitSelector8/1, 32BitSelector6/1, 32BitSelector1/1, 32BitSelector4/1, 32BitSelector3/1, 32BitSelector/1
  Demux7/1 -> Switch7/1
  Demux7/3 -> Terminator15/1
  Demux7/2 -> Terminator14/1
  Md57Calib/1 -> Demux7/1
  Md58Calib/1 -> Demux8/1
  Demux8/2 -> Terminator16/1
  Demux8/3 -> Terminator17/1
  Demux8/1 -> Switch8/1
  Md61Calib/1 -> Demux3/1
  Md62Calib/1 -> Demux2/1
  FamlyLCalib/1 -> Terminator_19/1
  FamlyRCalib/1 -> Terminator_20/1
  Demux9/3 -> Terminator19/1
  Md15Calib/1 -> Demux9/1
  Demux9/1 -> Switch9/1
  32BitSelector9/1 -> Switch9/2
  Demux9/2 -> Terminator18/1
  Constant/1 -> Switch9/3
  Switch9/1 -> Switch8/3

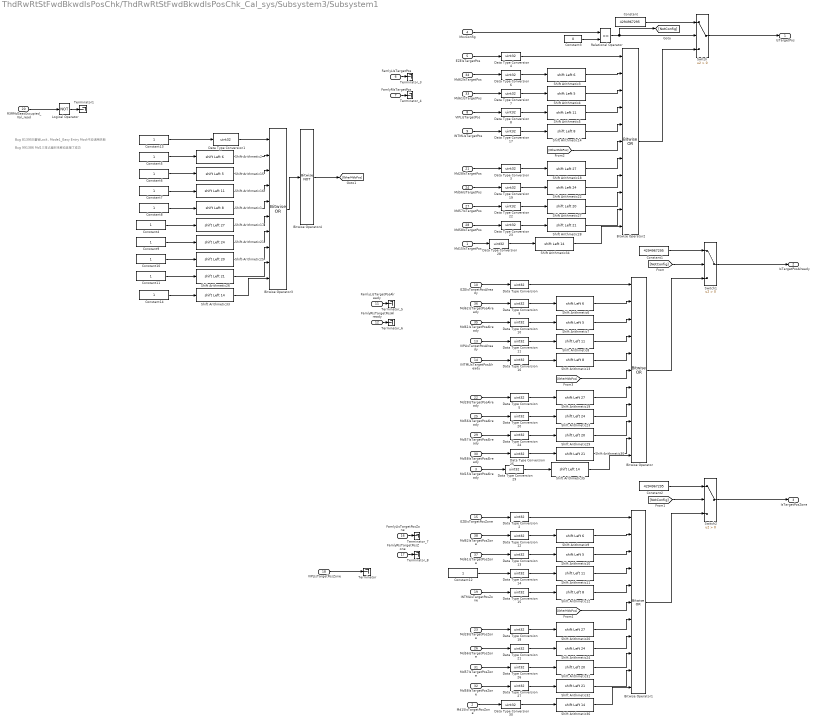
== system ThdRwRtStFwdBkwdIsPosChk/ThdRwRtStFwdBkwdIsPosChk_Cal_sys/Subsystem3/Subsystem1 ==
  note: Bug 991386 Md1 三排占座时未移动且报了成功
  note: Bug 813950 童锁Lock，Mode1_Easy Entry Mode 不应调用失败
  Md15IsTargetPos : Inport
  Md15IsTargetPosZone : Inport  Port=2
  Md15IsTargetPosAlready : Inport  Port=3
  MovConfig : Inport  Port=4
  EZEIsTargetPos : Inport  Port=5
  FamlyLIsTargetPos : Inport  Port=6
  FamlyRIsTargetPos : Inport  Port=7
  VIPLIsTargetPos : Inport  Port=8
  INTMLIsTargetPos : Inport  Port=9
  EZEIsTargetPosAlready : Inport  Port=10
  FamlyLIsTargetPosAlready : Inport  Port=11
  FamlyRIsTargetPosAlready : Inport  Port=12
  VIPLIsTargetPosAlready : Inport  Port=13
  INTMLIsTargetPosAlready : Inport  Port=14
  EZEIsTargetPosZone : Inport  Port=15
  FamlyLIsTargetPosZone : Inport  Port=16
  FamlyRIsTargetPosZone : Inport  Port=17
  VIPLIsTargetPosZone : Inport  Port=18
  INTMLIsTargetPosZone : Inport  Port=19
  R3RMdSeatOccupied_Val_read : Inport  Port=20
  Md28IsTargetPos : Inport  Port=21
  Md28IsTargetPosAlready : Inport  Port=22
  Md28IsTargetPosZone : Inport  Port=23
  Md56IsTargetPos : Inport  Port=24
  Md56IsTargetPosAlready : Inport  Port=25
  Md56IsTargetPosZone : Inport  Port=26
  Md57IsTargetPos : Inport  Port=27
  Md58IsTargetPos : Inport  Port=28
  Md57IsTargetPosAlready : Inport  Port=29
  Md58IsTargetPosAlready : Inport  Port=30
  Md57IsTargetPosZone : Inport  Port=31
  Md58IsTargetPosZone : Inport  Port=32
  Md61IsTargetPos : Inport  Port=33
  Md62IsTargetPos : Inport  Port=34
  Md61IsTargetPosAlready : Inport  Port=35
  Md62IsTargetPosAlready : Inport  Port=36
  Md61IsTargetPosZone : Inport  Port=37
  Md62IsTargetPosZone : Inport  Port=38
  Bitwise Operator : simulink/Logic and Bit Operations/Bitwise Operator  logicop=OR  UseBitMask=off  NumInputPorts=11  BitMask=bin2dec('11011001')  BitMaskRealWorld=Stored Integer
  Bitwise Operator1 : simulink/Logic and Bit Operations/Bitwise Operator  logicop=OR  UseBitMask=off  NumInputPorts=11  BitMask=bin2dec('11011001')  BitMaskRealWorld=Stored Integer
  Bitwise Operator2 : simulink/Logic and Bit Operations/Bitwise Operator  logicop=OR  UseBitMask=off  NumInputPorts=11  BitMask=bin2dec('11011001')  BitMaskRealWorld=Stored Integer
  Bitwise Operator3 : simulink/Logic and Bit Operations/Bitwise Operator  logicop=OR  UseBitMask=off  NumInputPorts=10  BitMask=bin2dec('11011001')  BitMaskRealWorld=Stored Integer
  Bitwise Operator4 : simulink/Logic and Bit Operations/Bitwise Operator  logicop=NOT  UseBitMask=off  BitMask=bin2dec('11011001')  BitMaskRealWorld=Stored Integer
  Constant : Constant  Value=4294967295  OutDataTypeStr=uint32
  Constant1 : Constant  Value=4294967295  OutDataTypeStr=uint32
  Constant{4..14} (11 alike) : Constant  OutDataTypeStr=uint32
  Constant2 : Constant  Value=4294967295  OutDataTypeStr=uint32
  Constant3 : Constant  Value=0  OutDataTypeStr=uint8
  Data Type Conversion{,1..30} (31 alike) : DataTypeConversion  OutDataTypeStr=uint32
  Logical Operator : Logic  Operator=NOT  AllPortsSameDT=off  OutDataTypeStr=boolean
  Relational Operator : RelationalOperator  Operator===  OutDataTypeStr=boolean  RndMeth=Simplest
  Shift Arithmetic{1,12..14} (4 alike) : ArithShift  BitShiftNumber=8  BitShiftDirection=Left
  Shift Arithmetic{4,7,10,15} (4 alike) : ArithShift  BitShiftNumber=5  BitShiftDirection=Left
  Shift Arithmetic{5,8,11,16} (4 alike) : ArithShift  BitShiftNumber=11  BitShiftDirection=Left
  Shift Arithmetic{17..20} (4 alike) : ArithShift  BitShiftNumber=27  BitShiftDirection=Left
  Shift Arithmetic{2..3,6,9} (4 alike) : ArithShift  BitShiftNumber=6  BitShiftDirection=Left
  Shift Arithmetic{21..24} (4 alike) : ArithShift  BitShiftNumber=24  BitShiftDirection=Left
  Shift Arithmetic{25,27,29,31} (4 alike) : ArithShift  BitShiftNumber=20  BitShiftDirection=Left
  Shift Arithmetic{26,28,30,32} (4 alike) : ArithShift  BitShiftNumber=21  BitShiftDirection=Left
  Shift Arithmetic{33..36} (4 alike) : ArithShift  BitShiftNumber=14  BitShiftDirection=Left
  Switch : Switch  Criteria=u2 > Threshold
  Switch1 : Switch  Criteria=u2 > Threshold
  Switch2 : Switch  Criteria=u2 > Threshold
  Terminator : Terminator
  Terminator1 : Terminator
  Terminator_{3..8} (6 alike) : Terminator
  IsTargetPos : Outport
      settings: EnsureOutportIsVirtual=on
  IsTargetPosAlready : Outport  Port=2
      settings: EnsureOutportIsVirtual=on
  IsTargetPosZone : Outport  Port=3
      settings: EnsureOutportIsVirtual=on
  wires:
  Constant3/1 -> Relational Operator/2
  Constant/1 -> Switch/1
  Relational Operator/1 -> [NotConfig], Switch/2
  MovConfig/1 -> Relational Operator/1
  Switch/1 -> IsTargetPos/1
  [NotConfig] -> Switch1/2
  Constant1/1 -> Switch1/1
  Switch1/1 -> IsTargetPosAlready/1
  Switch2/1 -> IsTargetPosZone/1
  Constant2/1 -> Switch2/1
  [NotConfig] -> Switch2/2
  Data Type Conversion/1 -> Bitwise Operator/1
  Data Type Conversion2/1 -> Bitwise Operator1/1
  Bitwise Operator1/1 -> Switch2/3
  Bitwise Operator/1 -> Switch1/3
  Data Type Conversion4/1 -> Bitwise Operator2/1
  Bitwise Operator2/1 -> Switch/3
  EZEIsTargetPos/1 -> Data Type Conversion4/1
  EZEIsTargetPosZone/1 -> Data Type Conversion2/1
  EZEIsTargetPosAlready/1 -> Data Type Conversion/1
  Shift Arithmetic3/1 -> Bitwise Operator2/2
  Shift Arithmetic4/1 -> Bitwise Operator2/3
  Shift Arithmetic5/1 -> Bitwise Operator2/4
  Data Type Conversion7/1 -> Shift Arithmetic4/1
  Data Type Conversion6/1 -> Shift Arithmetic3/1
  Data Type Conversion8/1 -> Shift Arithmetic5/1
  VIPLIsTargetPos/1 -> Data Type Conversion8/1
  VIPLIsTargetPosAlready/1 -> Data Type Conversion11/1
  Data Type Conversion11/1 -> Shift Arithmetic8/1
  Data Type Conversion9/1 -> Shift Arithmetic6/1
  Data Type Conversion10/1 -> Shift Arithmetic7/1
  Shift Arithmetic8/1 -> Bitwise Operator/4
  Shift Arithmetic7/1 -> Bitwise Operator/3
  Shift Arithmetic6/1 -> Bitwise Operator/2
  Data Type Conversion14/1 -> Shift Arithmetic11/1
  Data Type Conversion13/1 -> Shift Arithmetic10/1
  Shift Arithmetic10/1 -> Bitwise Operator1/3
  Shift Arithmetic9/1 -> Bitwise Operator1/2
  Shift Arithmetic11/1 -> Bitwise Operator1/4
  Data Type Conversion12/1 -> Shift Arithmetic9/1
  Data Type Conversion15/1 -> Shift Arithmetic12/1
  INTMLIsTargetPosZone/1 -> Data Type Conversion15/1
  Shift Arithmetic13/1 -> Bitwise Operator/5
  Data Type Conversion16/1 -> Shift Arithmetic13/1
  INTMLIsTargetPosAlready/1 -> Data Type Conversion16/1
  Shift Arithmetic14/1 -> Bitwise Operator2/5
  Data Type Conversion17/1 -> Shift Arithmetic14/1
  INTMLIsTargetPos/1 -> Data Type Conversion17/1
  Shift Arithmetic12/1 -> Bitwise Operator1/5
  Constant8/1 -> Shift Arithmetic1/1
  Shift Arithmetic1/1 -> Bitwise Operator3/5
  Constant7/1 -> Shift Arithmetic16/1
  Constant5/1 -> Shift Arithmetic2/1
  Constant6/1 -> Shift Arithmetic15/1
  Shift Arithmetic16/1 -> Bitwise Operator3/4
  Shift Arithmetic15/1 -> Bitwise Operator3/3
  Shift Arithmetic2/1 -> Bitwise Operator3/2
  Bitwise Operator3/1 -> Bitwise Operator4/1
  Bitwise Operator4/1 -> [OtherMdIsPos]
  [OtherMdIsPos] -> Bitwise Operator2/6
  [OtherMdIsPos] -> Bitwise Operator/6
  [OtherMdIsPos] -> Bitwise Operator1/6
  Data Type Conversion1/1 -> Bitwise Operator3/1
  R3RMdSeatOccupied_Val_read/1 -> Logical Operator/1
  Shift Arithmetic17/1 -> Bitwise Operator3/6
  Constant4/1 -> Shift Arithmetic17/1
  Md28IsTargetPos/1 -> Data Type Conversion3/1
  Data Type Conversion3/1 -> Shift Arithmetic18/1
  Shift Arithmetic18/1 -> Bitwise Operator2/7
  Shift Arithmetic19/1 -> Bitwise Operator/7
  Data Type Conversion5/1 -> Shift Arithmetic19/1
  Md28IsTargetPosAlready/1 -> Data Type Conversion5/1
  Md28IsTargetPosZone/1 -> Data Type Conversion18/1
  Data Type Conversion18/1 -> Shift Arithmetic20/1
  Shift Arithmetic20/1 -> Bitwise Operator1/7
  Constant9/1 -> Shift Arithmetic21/1
  Shift Arithmetic21/1 -> Bitwise Operator3/7
  Shift Arithmetic22/1 -> Bitwise Operator2/8
  Data Type Conversion19/1 -> Shift Arithmetic22/1
  Md56IsTargetPos/1 -> Data Type Conversion19/1
  Md56IsTargetPosAlready/1 -> Data Type Conversion20/1
  Data Type Conversion20/1 -> Shift Arithmetic23/1
  Shift Arithmetic23/1 -> Bitwise Operator/8
  Shift Arithmetic24/1 -> Bitwise Operator1/8
  Data Type Conversion21/1 -> Shift Arithmetic24/1
  Md56IsTargetPosZone/1 -> Data Type Conversion21/1
  Shift Arithmetic25/1 -> Bitwise Operator3/8
  Constant10/1 -> Shift Arithmetic25/1
  Constant11/1 -> Shift Arithmetic26/1
  Shift Arithmetic26/1 -> Bitwise Operator3/9
  Md57IsTargetPos/1 -> Data Type Conversion22/1
  Data Type Conversion22/1 -> Shift Arithmetic27/1
  Shift Arithmetic27/1 -> Bitwise Operator2/9
  Shift Arithmetic28/1 -> Bitwise Operator2/10
  Data Type Conversion23/1 -> Shift Arithmetic28/1
  Md58IsTargetPos/1 -> Data Type Conversion23/1
  Shift Arithmetic29/1 -> Bitwise Operator/9
  Data Type Conversion24/1 -> Shift Arithmetic29/1
  Md57IsTargetPosAlready/1 -> Data Type Conversion24/1
  Md58IsTargetPosAlready/1 -> Data Type Conversion25/1
  Data Type Conversion25/1 -> Shift Arithmetic30/1
  Shift Arithmetic30/1 -> Bitwise Operator/10
  Md57IsTargetPosZone/1 -> Data Type Conversion26/1
  Data Type Conversion26/1 -> Shift Arithmetic31/1
  Shift Arithmetic31/1 -> Bitwise Operator1/9
  Shift Arithmetic32/1 -> Bitwise Operator1/10
  Data Type Conversion27/1 -> Shift Arithmetic32/1
  Md58IsTargetPosZone/1 -> Data Type Conversion27/1
  Constant12/1 -> Data Type Conversion14/1
  VIPLIsTargetPosZone/1 -> Terminator/1
  Logical Operator/1 -> Terminator1/1
  Constant13/1 -> Data Type Conversion1/1
  Md61IsTargetPos/1 -> Data Type Conversion7/1
  Md62IsTargetPos/1 -> Data Type Conversion6/1
  Md61IsTargetPosAlready/1 -> Data Type Conversion10/1
  Md62IsTargetPosAlready/1 -> Data Type Conversion9/1
  Md61IsTargetPosZone/1 -> Data Type Conversion13/1
  Md62IsTargetPosZone/1 -> Data Type Conversion12/1
  FamlyLIsTargetPos/1 -> Terminator_3/1
  FamlyRIsTargetPos/1 -> Terminator_4/1
  FamlyLIsTargetPosAlready/1 -> Terminator_5/1
  FamlyRIsTargetPosAlready/1 -> Terminator_6/1
  FamlyLIsTargetPosZone/1 -> Terminator_7/1
  FamlyRIsTargetPosZone/1 -> Terminator_8/1
  Constant14/1 -> Shift Arithmetic33/1
  Shift Arithmetic33/1 -> Bitwise Operator3/10
  Data Type Conversion28/1 -> Shift Arithmetic34/1
  Shift Arithmetic34/1 -> Bitwise Operator2/11
  Md15IsTargetPos/1 -> Data Type Conversion28/1
  Data Type Conversion29/1 -> Shift Arithmetic35/1
  Shift Arithmetic35/1 -> Bitwise Operator/11
  Md15IsTargetPosAlready/1 -> Data Type Conversion29/1
  Data Type Conversion30/1 -> Shift Arithmetic36/1
  Md15IsTargetPosZone/1 -> Data Type Conversion30/1
  Shift Arithmetic36/1 -> Bitwise Operator1/11

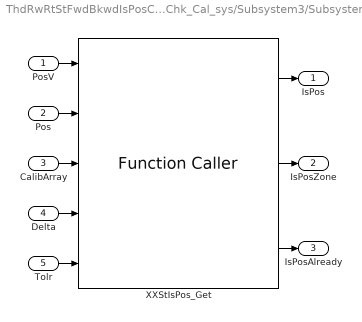
== system ThdRwRtStFwdBkwdIsPosChk/ThdRwRtStFwdBkwdIsPosChk_Cal_sys/Subsystem3/Subsystem10 ==
  PosV : Inport
  Pos : Inport  Port=2
  CalibArray : Inport  Port=3
  Delta : Inport  Port=4
  Tolr : Inport  Port=5
  XXStIsPos_Get : FunctionCaller  FunctionPrototype=[IsPos,IsPosZone,IsPosAlready] = XXStIsPos_Get(PosV,Pos,CalibArray,Delta,Tolr)  InputArgumentSpecifications=boolean(true), uint16(1), uint16([1;1;1]), uint16(1), uint16(1)  OutputArgumentSpecifications=boolean(true), boolean(true), boolean(true)
  IsPos : Outport
  IsPosZone : Outport  Port=2
  IsPosAlready : Outport  Port=3
  wires:
  Pos/1 -> XXStIsPos_Get/2
  Delta/1 -> XXStIsPos_Get/4
  CalibArray/1 -> XXStIsPos_Get/3
  XXStIsPos_Get/2 -> IsPosZone/1
  XXStIsPos_Get/1 -> IsPos/1
  Tolr/1 -> XXStIsPos_Get/5
  XXStIsPos_Get/3 -> IsPosAlready/1
  PosV/1 -> XXStIsPos_Get/1

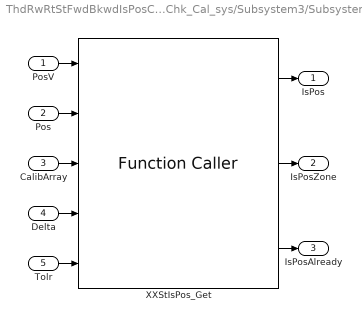
== system ThdRwRtStFwdBkwdIsPosChk/ThdRwRtStFwdBkwdIsPosChk_Cal_sys/Subsystem3/Subsystem11 ==
  PosV : Inport
  Pos : Inport  Port=2
  CalibArray : Inport  Port=3
  Delta : Inport  Port=4
  Tolr : Inport  Port=5
  XXStIsPos_Get : FunctionCaller  FunctionPrototype=[IsPos,IsPosZone,IsPosAlready] = XXStIsPos_Get(PosV,Pos,CalibArray,Delta,Tolr)  InputArgumentSpecifications=boolean(true), uint16(1), uint16([1;1;1]), uint16(1), uint16(1)  OutputArgumentSpecifications=boolean(true), boolean(true), boolean(true)
  IsPos : Outport
  IsPosZone : Outport  Port=2
  IsPosAlready : Outport  Port=3
  wires:
  PosV/1 -> XXStIsPos_Get/1
  XXStIsPos_Get/3 -> IsPosAlready/1
  Tolr/1 -> XXStIsPos_Get/5
  XXStIsPos_Get/1 -> IsPos/1
  XXStIsPos_Get/2 -> IsPosZone/1
  CalibArray/1 -> XXStIsPos_Get/3
  Delta/1 -> XXStIsPos_Get/4
  Pos/1 -> XXStIsPos_Get/2

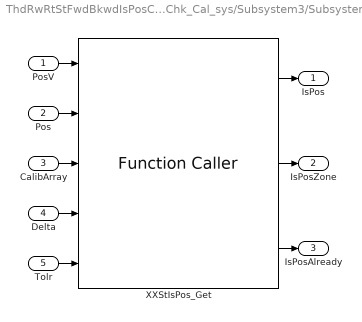
== system ThdRwRtStFwdBkwdIsPosChk/ThdRwRtStFwdBkwdIsPosChk_Cal_sys/Subsystem3/Subsystem12 ==
  PosV : Inport
  Pos : Inport  Port=2
  CalibArray : Inport  Port=3
  Delta : Inport  Port=4
  Tolr : Inport  Port=5
  XXStIsPos_Get : FunctionCaller  FunctionPrototype=[IsPos,IsPosZone,IsPosAlready] = XXStIsPos_Get(PosV,Pos,CalibArray,Delta,Tolr)  InputArgumentSpecifications=boolean(true), uint16(1), uint16([1;1;1]), uint16(1), uint16(1)  OutputArgumentSpecifications=boolean(true), boolean(true), boolean(true)
  IsPos : Outport
  IsPosZone : Outport  Port=2
  IsPosAlready : Outport  Port=3
  wires:
  Pos/1 -> XXStIsPos_Get/2
  Delta/1 -> XXStIsPos_Get/4
  CalibArray/1 -> XXStIsPos_Get/3
  XXStIsPos_Get/2 -> IsPosZone/1
  XXStIsPos_Get/1 -> IsPos/1
  Tolr/1 -> XXStIsPos_Get/5
  XXStIsPos_Get/3 -> IsPosAlready/1
  PosV/1 -> XXStIsPos_Get/1

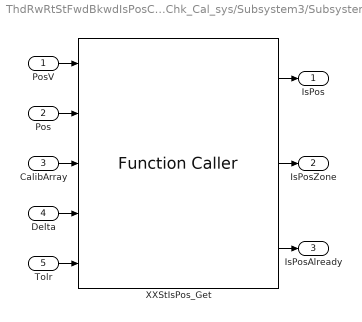
== system ThdRwRtStFwdBkwdIsPosChk/ThdRwRtStFwdBkwdIsPosChk_Cal_sys/Subsystem3/Subsystem13 ==
  PosV : Inport
  Pos : Inport  Port=2
  CalibArray : Inport  Port=3
  Delta : Inport  Port=4
  Tolr : Inport  Port=5
  XXStIsPos_Get : FunctionCaller  FunctionPrototype=[IsPos,IsPosZone,IsPosAlready] = XXStIsPos_Get(PosV,Pos,CalibArray,Delta,Tolr)  InputArgumentSpecifications=boolean(true), uint16(1), uint16([1;1;1]), uint16(1), uint16(1)  OutputArgumentSpecifications=boolean(true), boolean(true), boolean(true)
  IsPos : Outport
  IsPosZone : Outport  Port=2
  IsPosAlready : Outport  Port=3
  wires:
  PosV/1 -> XXStIsPos_Get/1
  XXStIsPos_Get/3 -> IsPosAlready/1
  Tolr/1 -> XXStIsPos_Get/5
  XXStIsPos_Get/1 -> IsPos/1
  XXStIsPos_Get/2 -> IsPosZone/1
  CalibArray/1 -> XXStIsPos_Get/3
  Delta/1 -> XXStIsPos_Get/4
  Pos/1 -> XXStIsPos_Get/2

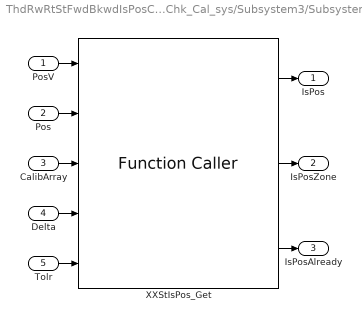
== system ThdRwRtStFwdBkwdIsPosChk/ThdRwRtStFwdBkwdIsPosChk_Cal_sys/Subsystem3/Subsystem14 ==
  PosV : Inport
  Pos : Inport  Port=2
  CalibArray : Inport  Port=3
  Delta : Inport  Port=4
  Tolr : Inport  Port=5
  XXStIsPos_Get : FunctionCaller  FunctionPrototype=[IsPos,IsPosZone,IsPosAlready] = XXStIsPos_Get(PosV,Pos,CalibArray,Delta,Tolr)  InputArgumentSpecifications=boolean(true), uint16(1), uint16([1;1;1]), uint16(1), uint16(1)  OutputArgumentSpecifications=boolean(true), boolean(true), boolean(true)
  IsPos : Outport
  IsPosZone : Outport  Port=2
  IsPosAlready : Outport  Port=3
  wires:
  PosV/1 -> XXStIsPos_Get/1
  XXStIsPos_Get/3 -> IsPosAlready/1
  Tolr/1 -> XXStIsPos_Get/5
  XXStIsPos_Get/1 -> IsPos/1
  XXStIsPos_Get/2 -> IsPosZone/1
  CalibArray/1 -> XXStIsPos_Get/3
  Delta/1 -> XXStIsPos_Get/4
  Pos/1 -> XXStIsPos_Get/2

== system ThdRwRtStFwdBkwdIsPosChk/ThdRwRtStFwdBkwdIsPosChk_Cal_sys/Subsystem3/Subsystem2 ==
  CmdSrv : Inport
  Logical Operator : Logic  Operator=NOT  AllPortsSameDT=off  OutDataTypeStr=boolean
  IsTargetPos : Outport
  wires:
  Logical Operator/1 -> IsTargetPos/1
  CmdSrv/1 -> Logical Operator/1

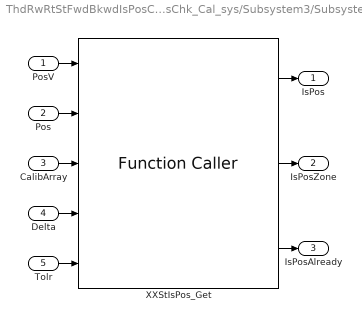
== system ThdRwRtStFwdBkwdIsPosChk/ThdRwRtStFwdBkwdIsPosChk_Cal_sys/Subsystem3/Subsystem3 ==
  PosV : Inport
  Pos : Inport  Port=2
  CalibArray : Inport  Port=3
  Delta : Inport  Port=4
  Tolr : Inport  Port=5
  XXStIsPos_Get : FunctionCaller  FunctionPrototype=[IsPos,IsPosZone,IsPosAlready] = XXStIsPos_Get(PosV,Pos,CalibArray,Delta,Tolr)  InputArgumentSpecifications=boolean(true), uint16(1), uint16([1;1;1]), uint16(1), uint16(1)  OutputArgumentSpecifications=boolean(true), boolean(true), boolean(true)
  IsPos : Outport
  IsPosZone : Outport  Port=2
  IsPosAlready : Outport  Port=3
  wires:
  PosV/1 -> XXStIsPos_Get/1
  XXStIsPos_Get/3 -> IsPosAlready/1
  Tolr/1 -> XXStIsPos_Get/5
  XXStIsPos_Get/1 -> IsPos/1
  XXStIsPos_Get/2 -> IsPosZone/1
  CalibArray/1 -> XXStIsPos_Get/3
  Delta/1 -> XXStIsPos_Get/4
  Pos/1 -> XXStIsPos_Get/2

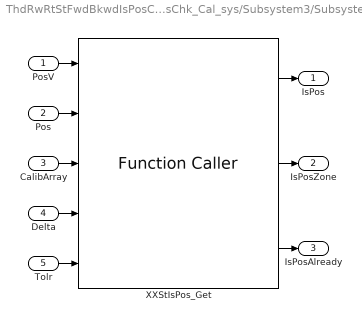
== system ThdRwRtStFwdBkwdIsPosChk/ThdRwRtStFwdBkwdIsPosChk_Cal_sys/Subsystem3/Subsystem4 ==
  PosV : Inport
  Pos : Inport  Port=2
  CalibArray : Inport  Port=3
  Delta : Inport  Port=4
  Tolr : Inport  Port=5
  XXStIsPos_Get : FunctionCaller  FunctionPrototype=[IsPos,IsPosZone,IsPosAlready] = XXStIsPos_Get(PosV,Pos,CalibArray,Delta,Tolr)  InputArgumentSpecifications=boolean(true), uint16(1), uint16([1;1;1]), uint16(1), uint16(1)  OutputArgumentSpecifications=boolean(true), boolean(true), boolean(true)
  IsPos : Outport
  IsPosZone : Outport  Port=2
  IsPosAlready : Outport  Port=3
  wires:
  PosV/1 -> XXStIsPos_Get/1
  XXStIsPos_Get/3 -> IsPosAlready/1
  Tolr/1 -> XXStIsPos_Get/5
  XXStIsPos_Get/1 -> IsPos/1
  XXStIsPos_Get/2 -> IsPosZone/1
  CalibArray/1 -> XXStIsPos_Get/3
  Delta/1 -> XXStIsPos_Get/4
  Pos/1 -> XXStIsPos_Get/2

== system ThdRwRtStFwdBkwdIsPosChk/ThdRwRtStFwdBkwdIsPosChk_Cal_sys/Subsystem3/Subsystem5 ==
  PosV : Inport
  Pos : Inport  Port=2
  CalibArray : Inport  Port=3
  Delta : Inport  Port=4
  Tolr : Inport  Port=5
  XXStIsPos_Get : FunctionCaller  FunctionPrototype=[IsPos,IsPosZone,IsPosAlready] = XXStIsPos_Get(PosV,Pos,CalibArray,Delta,Tolr)  InputArgumentSpecifications=boolean(true), uint16(1), uint16([1;1;1]), uint16(1), uint16(1)  OutputArgumentSpecifications=boolean(true), boolean(true), boolean(true)
  IsPos : Outport
  IsPosZone : Outport  Port=2
  IsPosAlready : Outport  Port=3
  wires:
  PosV/1 -> XXStIsPos_Get/1
  XXStIsPos_Get/3 -> IsPosAlready/1
  Tolr/1 -> XXStIsPos_Get/5
  XXStIsPos_Get/1 -> IsPos/1
  XXStIsPos_Get/2 -> IsPosZone/1
  CalibArray/1 -> XXStIsPos_Get/3
  Delta/1 -> XXStIsPos_Get/4
  Pos/1 -> XXStIsPos_Get/2

== system ThdRwRtStFwdBkwdIsPosChk/ThdRwRtStFwdBkwdIsPosChk_Cal_sys/Subsystem3/Subsystem6 ==
  PosV : Inport
  Pos : Inport  Port=2
  CalibArray : Inport  Port=3
  Delta : Inport  Port=4
  Tolr : Inport  Port=5
  XXStIsPos_Get : FunctionCaller  FunctionPrototype=[IsPos,IsPosZone,IsPosAlready] = XXStIsPos_Get(PosV,Pos,CalibArray,Delta,Tolr)  InputArgumentSpecifications=boolean(true), uint16(1), uint16([1;1;1]), uint16(1), uint16(1)  OutputArgumentSpecifications=boolean(true), boolean(true), boolean(true)
  IsPos : Outport
  IsPosZone : Outport  Port=2
  IsPosAlready : Outport  Port=3
  wires:
  PosV/1 -> XXStIsPos_Get/1
  XXStIsPos_Get/3 -> IsPosAlready/1
  Tolr/1 -> XXStIsPos_Get/5
  XXStIsPos_Get/1 -> IsPos/1
  XXStIsPos_Get/2 -> IsPosZone/1
  CalibArray/1 -> XXStIsPos_Get/3
  Delta/1 -> XXStIsPos_Get/4
  Pos/1 -> XXStIsPos_Get/2

== system ThdRwRtStFwdBkwdIsPosChk/ThdRwRtStFwdBkwdIsPosChk_Cal_sys/Subsystem3/Subsystem7 ==
  PosV : Inport
  Pos : Inport  Port=2
  CalibArray : Inport  Port=3
  Delta : Inport  Port=4
  Tolr : Inport  Port=5
  XXStIsPos_Get : FunctionCaller  FunctionPrototype=[IsPos,IsPosZone,IsPosAlready] = XXStIsPos_Get(PosV,Pos,CalibArray,Delta,Tolr)  InputArgumentSpecifications=boolean(true), uint16(1), uint16([1;1;1]), uint16(1), uint16(1)  OutputArgumentSpecifications=boolean(true), boolean(true), boolean(true)
  IsPos : Outport
  IsPosZone : Outport  Port=2
  IsPosAlready : Outport  Port=3
  wires:
  Pos/1 -> XXStIsPos_Get/2
  Delta/1 -> XXStIsPos_Get/4
  CalibArray/1 -> XXStIsPos_Get/3
  XXStIsPos_Get/2 -> IsPosZone/1
  XXStIsPos_Get/1 -> IsPos/1
  Tolr/1 -> XXStIsPos_Get/5
  XXStIsPos_Get/3 -> IsPosAlready/1
  PosV/1 -> XXStIsPos_Get/1
